simulink subsystem "PieroControladoZ"  (R2023b)
settings: Solver=VariableStepAuto  StartTime=0.0  StopTime=10.0  RelTol=1e-3
settings Model: Creator=Carlos  LastModifiedBy=Carlos

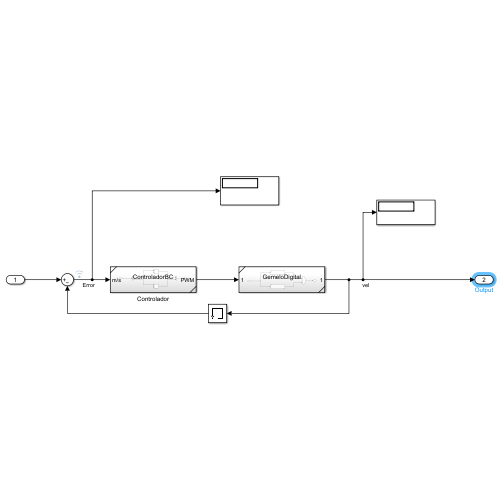
[thumbnail: Simulink's stored preview of the top-level diagram]
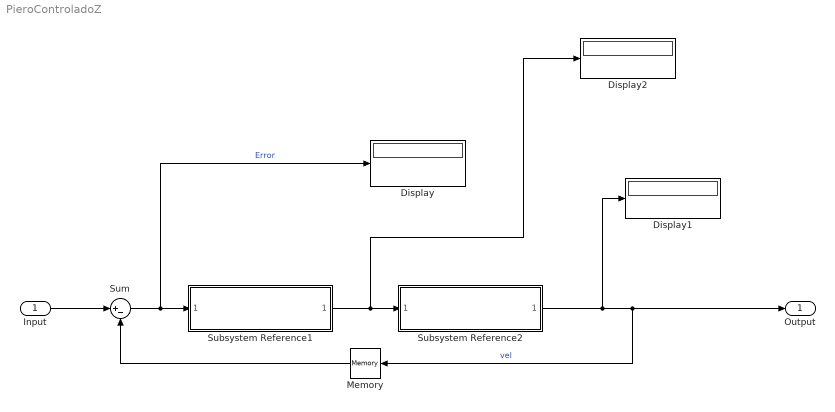
== system PieroControladoZ ==
  Input : Inport  OutDataTypeStr=double
  Display : Display
  Display1 : Display
  Display2 : Display
  Memory : Memory
  Subsystem Reference1 : Subsystem  ReferencedSubsystem=ControladorBCZ
  Subsystem Reference2 : Subsystem  ReferencedSubsystem=GemeloDigitalZ
  Sum : Sum  Inputs=|+-
  Output : Outport  OutDataTypeStr=double
  wires:
  Memory/1 -> Sum/2
  Sum/1 -> Display/1, Subsystem Reference1/1  "Error"
  Subsystem Reference2/1 -> Display1/1, Output/1, Memory/1  "vel"
  Subsystem Reference1/1 -> Subsystem Reference2/1, Display2/1
  Input/1 -> Sum/1
